simulink model "control_on_off"  (R2020a)
settings: Solver=VariableStepAuto  StartTime=0.0  StopTime=800  RelTol=1e-3
values from neighbouring files (symbols this model uses):
  DEN1 = [102 1]    [lab5.m]
  Dtime1 = 0.5    [lab5.m]
  NUM1 = [32.74]    [lab5.m]
settings Model: Creator=Gloria Dani Abe  LastModifiedBy=Gloria Dani Abe

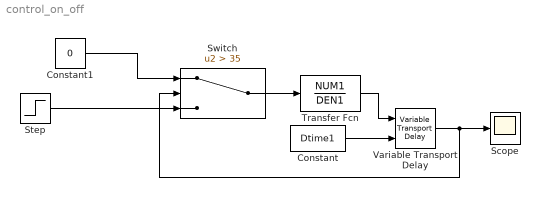
== system control_on_off ==
  Constant : Constant  Value=Dtime1
  Constant1 : Constant  Value=0
  Scope : Scope
  Step : Step  SampleTime=0
  Switch : Switch  Criteria=u2 > Threshold  Threshold=35
  Transfer Fcn : TransferFcn  Numerator=NUM1  Denominator=DEN1
  Variable Transport Delay : VariableTransportDelay  VariableDelayType=Variable transport delay  MaximumDelay=10
  wires:
  Constant/1 -> Variable Transport Delay/2
  Switch/1 -> Transfer Fcn/1
  Transfer Fcn/1 -> Variable Transport Delay/1
  Variable Transport Delay/1 -> Scope/1, Switch/2
  Step/1 -> Switch/3
  Constant1/1 -> Switch/1
